simulink subsystem "MPC5_nlpsol"  (R2023b)
settings: Solver=VariableStepAuto  StartTime=0.0  StopTime=10.0  RelTol=1e-3
undefined symbols (not defined in the file): param_FeasibleBlock_init_guess, param_MPC5, param_MPC5_init_guess, param_traj_data, param_weight_init
settings Model: Creator=emu  LastModifiedBy=emu

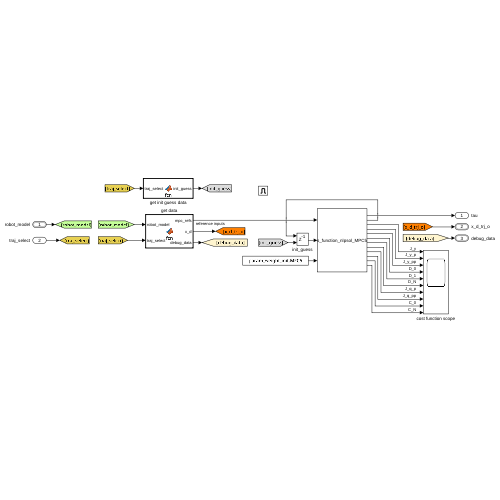
[thumbnail: Simulink's stored preview of the top-level diagram]
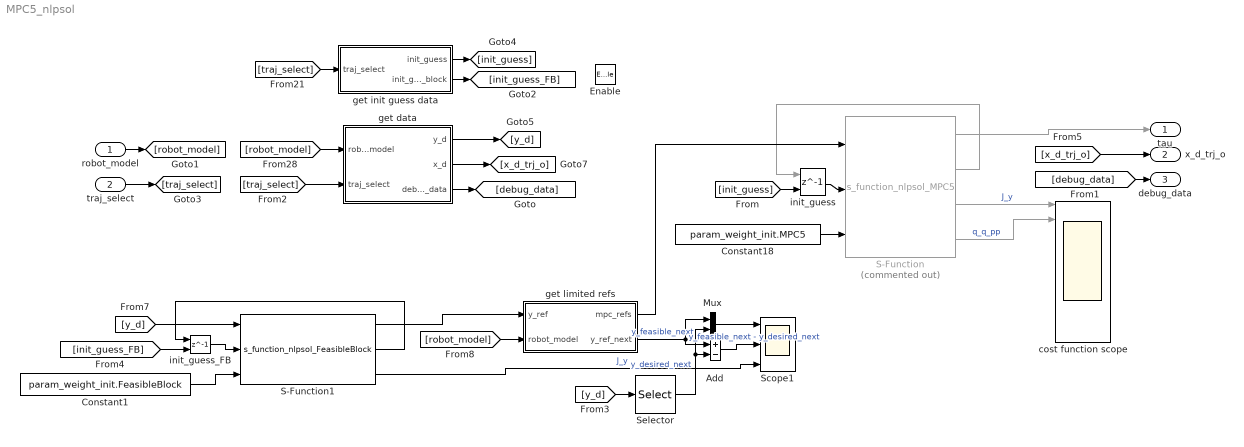
== system MPC5_nlpsol ==
  robot_model : Inport  OutDataTypeStr=Bus: robot_model
  traj_select : Inport  Port=2
  Enable : EnablePort
  Add : Sum  Inputs=+-
  Constant1 : Constant  Value=param_weight_init.FeasibleBlock  VectorParams1D=off
  Constant18 : Constant  Value=param_weight_init.MPC5  VectorParams1D=off
  Mux : Mux  Inputs=2
  S-Function : S-Function  Commented=on  FunctionName=s_function_nlpsol_MPC5  Parameters='s_functions/MPC5.casadi', 'MPC5'  SFunctionDeploymentMode=off  EnableBusSupport=off
  S-Function1 : S-Function  FunctionName=s_function_nlpsol_FeasibleBlock  Parameters='s_functions/FeasibleBlock.casadi', 'FeasibleBlock'  SFunctionDeploymentMode=off  EnableBusSupport=off
  Scope1 : Scope  NumInputPorts=3
  Selector : Selector  InputPortWidth=12  IndexOptions=Index vector (dialog)  Indices=[1:2]  OutputSizes=1
  cost function scope : Scope  NumInputPorts=10
  get data : MATLAB Function  TreatAsAtomicUnit=on
  get init guess data : MATLAB Function  TreatAsAtomicUnit=on
  get limited refs : MATLAB Function  TreatAsAtomicUnit=on
  init_guess : Delay  DelayLength=1  InitialConditionSource=Input port  InitialCondition=1
      settings: InputPortMap=u0,p4
  init_guess_FB : Delay  DelayLength=1  InitialConditionSource=Input port  InitialCondition=1
      settings: InputPortMap=u0,p4
  tau : Outport
  x_d_trj_o : Outport  Port=2  OutDataTypeStr=Bus: x_d
  debug_data : Outport  Port=3  OutDataTypeStr=Bus: debug_data_bus
  wires:
  [init_guess] -> init_guess/2
  get init guess data/1(init_guess) -> [init_guess]
  [traj_select] -> get data/2(traj_select)
  [robot_model] -> get data/1(robot_model)
  S-Function/2 -> init_guess/1
  [debug_data] -> debug_data/1
  init_guess/1 -> S-Function/2
  S-Function/4 -> cost function scope/2  "q_q_pp"
  [traj_select] -> get init guess data/1(traj_select)
  traj_select/1 -> [traj_select]
  S-Function/1 -> tau/1
  get data/2(x_d) -> [x_d_trj_o]
  get data/3(debug_data) -> [debug_data]
  robot_model/1 -> [robot_model]
  [x_d_trj_o] -> x_d_trj_o/1
  S-Function/3 -> cost function scope/1  "J_y"
  Constant18/1 -> S-Function/3
  Selector/1 -> Mux/2, Add/2  "y_desired_next"
  [robot_model] -> get limited refs/2(robot_model)
  S-Function1/3 -> Scope1/3  "J_y"
  [y_d] -> Selector/1
  init_guess_FB/1 -> S-Function1/2
  Constant1/1 -> S-Function1/3
  [init_guess_FB] -> init_guess_FB/2
  Mux/1 -> Scope1/1
  get limited refs/2(y_ref_next) -> Add/1, Mux/1  "y_feasible_next"
  S-Function1/2 -> init_guess_FB/1
  Add/1 -> Scope1/2  "y_feasible_next - y_desired_next"
  [y_d] -> S-Function1/1
  S-Function1/1 -> get limited refs/1(y_ref)
  get data/1(y_d) -> [y_d]
  get limited refs/1(mpc_refs) -> S-Function/1
  get init guess data/2(init_guess_feasible_block) -> [init_guess_FB]

== matlab function MPC5_nlpsol/get data ==
  settings: updateMethod=DISCRETE  sampleTime=param_global.Ta
  data: y_d output; robot_model input Bus: robot_model; param_MPC5 parameter; x_d output Bus: x_d; debug_data output Bus: debug_data_bus; param_traj_data parameter; traj_select input
function [y_d, x_d, debug_data] = fcn(robot_model, param_MPC5, param_traj_data, traj_select)
persistent cnt;

if(isempty(cnt))
    cnt = 1;
end

param_MPC = param_MPC5;
N         = param_MPC.N;
N_step    = param_MPC.N_step;

% Parameters
%q    = robot_model.q;      % generalized coordinates
q_p  = robot_model.q_p;  % time derivative of generalized coordinates
q_pp = robot_model.q_pp;
H    = robot_model.H;
J    = robot_model.J;
J_p  = robot_model.J_p;

% Current Pose of Endeffector
p = H(1:2,4);
p_p = J(1:2,1:2)*q_p;
p_pp = J(1:2,1:2)*q_pp + J_p(1:2,1:2)*q_p;

R = H(1:3,1:3);

% desired Orientation as Rotationmatrix
q_e = rotation2quaternion(R);

% Error of Position (translation) and first time derivative
q_err = quat_mult(q_e, quat_inv(param_traj_data.q_d(1:4, cnt, traj_select)));

% Assemble vector of recieved output measurements
p_d_traj    = param_traj_data.p_d(   1:3, cnt : N_step : cnt + (N  )*N_step, traj_select);
p_d_p_traj  = param_traj_data.p_d_p( 1:3, cnt : N_step : cnt + (N  )*N_step, traj_select);
p_d_pp_traj = param_traj_data.p_d_pp(1:3, cnt : N_step : cnt + (N-1)*N_step, traj_select);

y_ref    = p_d_traj(   1:2, 1 + (0:N  ) ); %       y1,   y2,   ... yN
%y_ref_p  = p_d_p_traj( 1:2, 1 + (1:N  ) ); %       y1p,  y2p,  ... yNp
%y_ref_pp = p_d_pp_traj(1:2, 1 + (0:N-1) ); % y0pp, y1pp, y2pp, ... yN-1pp

cnt = cnt+1;

%% Reference out

y_d = y_ref(:)';

%% TRAJECTORY OUT
x_d.p_d       = p_d_traj(1:3,1);    %y0
x_d.p_d_p     = p_d_p_traj(1:3,1);  %y0p
x_d.p_d_pp    = p_d_pp_traj(1:3,1); %y0pp
x_d.q_d       = [0; 0; 0; 0];
x_d.omega_d   = [0; 0; 0];
x_d.omega_d_p = [0; 0; 0];

%% DEBUG
debug_data.p    = p(1:2);
debug_data.p_p  = p_p(1:2);
debug_data.p_pp = p_pp(1:2);
debug_data.rot_x_err = q_err(2);
debug_data.rot_y_err = q_err(3);
debug_data.rot_z_err = q_err(4);

== matlab function MPC5_nlpsol/get limited refs ==
  data: y_ref input; robot_model input; mpc_refs output; param_robot parameter; y_ref_next output
function [mpc_refs, y_ref_next] = fcn(y_ref, robot_model, param_robot)
    q    = robot_model.q;      % generalized coordinates
    q_p  = robot_model.q_p;  % time derivative of generalized coordinates

    x_k = [q;q_p];

    mpc_refs = [x_k(:); y_ref(:)]';
    y_ref_next = y_ref(1:2)';
end

== matlab function MPC5_nlpsol/get init guess data ==
  data: traj_select input; param_MPC5_init_guess parameter; init_guess output; init_guess_feasible_block output; param_FeasibleBlock_init_guess parameter
function [init_guess,init_guess_feasible_block]  = fcn(traj_select, param_MPC5_init_guess, param_FeasibleBlock_init_guess)

init_guess = param_MPC5_init_guess.init_guess(traj_select,:);
init_guess_feasible_block = param_FeasibleBlock_init_guess.init_guess(traj_select,:);
